simulink model "Cruise_Control_With_PID_Cont"  (R2020b)
settings: Solver=ode45  StartTime=0.0  StopTime=120  RelTol=1e-3
values from neighbouring files (symbols this model uses):
  b = 50.0    [Data1.sldd]    (also in data.mat = 50)
  m = 1000.0    [Data1.sldd]    (also in data.mat = 1000)
settings Model: DataDictionary=Data1.sldd  Creator=vijay jagtap  LastModifiedBy=vijay jagtap
settings SolverCC: MaxConsecutiveMinStep=1000
settings DataIOCC: SaveOutput=off  SaveTime=off

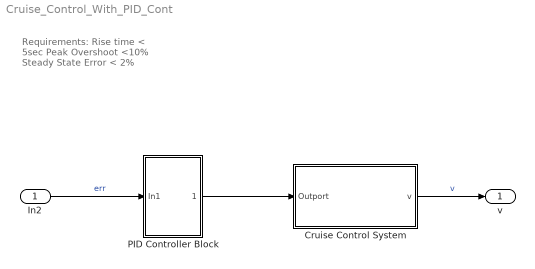
== system Cruise_Control_With_PID_Cont ==
  note: Requirements:
      |
      | Rise time < 5sec
      | Peak Overshoot <10%
      | Steady State Error < 2%
  In2 : Inport  OutDataTypeStr=double  PortDimensions=1  SampleTime=0
  Cruise Control System : Subsystem
  PID Controller Block : Subsystem  mask{Kp=490, Ki=70, Kd=260}
  v : Outport  OutDataTypeStr=double  PortDimensions=1  SampleTime=0
  wires:
  In2/1 -> PID Controller Block/1(In1)  "err"
  PID Controller Block/1(Outport) -> Cruise Control System/1(Outport)
  Cruise Control System/1(v) -> v/1  "v"

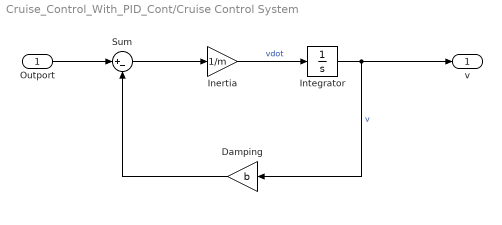
== system Cruise_Control_With_PID_Cont/Cruise Control System ==
  Outport : Inport
  Damping : Gain  Gain=b
  Inertia : Gain  Gain=1/m
  Integrator : Integrator
  Sum : Sum  Inputs=|+-
  v : Outport
  wires:
  Inertia/1 -> Integrator/1  "vdot"
  Integrator/1 -> v/1, Damping/1  "v"
  Damping/1 -> Sum/2
  Sum/1 -> Inertia/1
  Outport/1 -> Sum/1

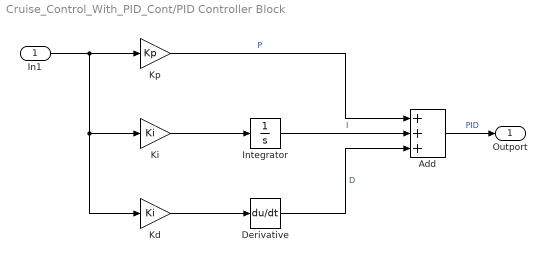
== system Cruise_Control_With_PID_Cont/PID Controller Block ==
  In1 : Inport
  Add : Sum  Inputs=+++
  Derivative : Derivative
  Integrator : Integrator
  Kd : Gain  Gain=Ki
  Ki : Gain  Gain=Ki
  Kp : Gain  Gain=Kp
  Outport : Outport
  wires:
  In1/1 -> Kd/1, Ki/1, Kp/1
  Kd/1 -> Derivative/1
  Kp/1 -> Add/1  "P"
  Ki/1 -> Integrator/1
  Derivative/1 -> Add/3  "D"
  Integrator/1 -> Add/2  "I"
  Add/1 -> Outport/1  "PID"
